simulink model "Hacheur_4_quadrant"  (R2013a)
settings: Solver=ode1  StartTime=0.0  StopTime=10  FixedStep=1e-5  RelTol=1e-3
undefined symbols (not defined in the file or in its folder): Tmli
libraries: powerlib x10, simulink x1
settings Model: Creator=hp  LastModifiedBy=hp
settings DataIOCC: InspectSignalLogs=on

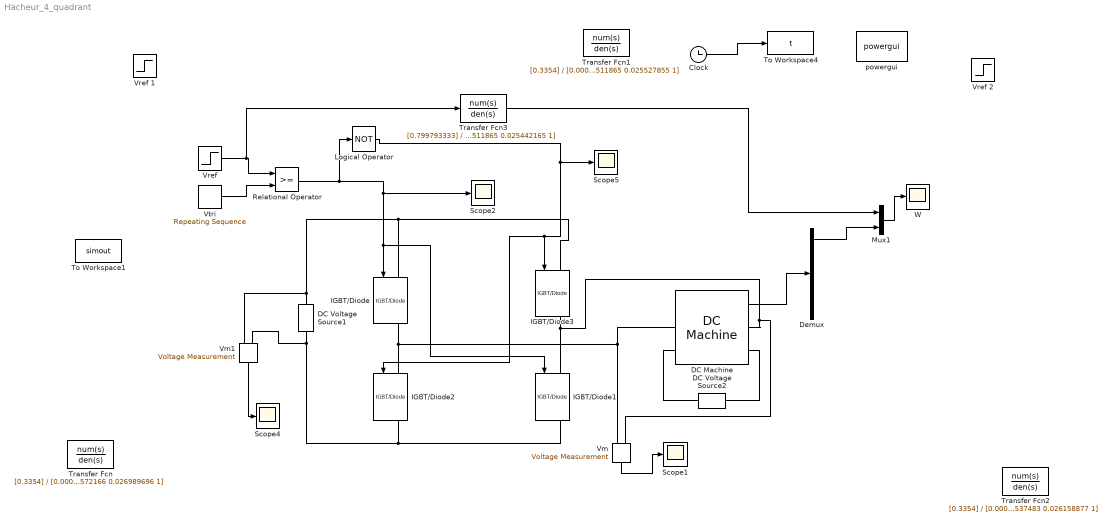
== system Hacheur_4_quadrant ==
  Clock : Clock
  DC Machine : powerlib/Machines/DC Machine  PresetModel=02: 5HP 240V 1750RPM Field:150V  MechanicalLoad=Torque TL  FieldType=Wound  ShowDetailedParameters=on  RLa=[0.78 0.016]  RLf=[150 112.5]  Laf=1.234  MachineConstant=Torque constant (N.m/A)  Ke=1.8  Kt=1.8  J=0.05  Bm=0.01  Tf=0  w0=1  Ifinit=1  TsPowergui=0  TsBlock=-1
  DC Voltage Source1 : powerlib/Electrical Sources/DC Voltage Source  Amplitude=240  Measurements=None
  DC Voltage Source2 : powerlib/Electrical Sources/DC Voltage Source  Amplitude=150  Measurements=None
  Demux : Demux
  IGBT/Diode{,1..3} (4 alike) : powerlib/Power Electronics/IGBT//Diode  Ron=1e-3  Rs=1e5  Cs=inf  Measurements=on
  Logical Operator : Logic  Operator=NOT  AllPortsSameDT=off  OutDataTypeStr=boolean
  Mux1 : Mux  Inputs=2
  Relational Operator : RelationalOperator  OutDataTypeStr=boolean
  Scope{1..2,4..5} (4 alike) : Scope
      Scope4 settings: SaveName=ScopeData3
      Scope5 settings: SaveName=ScopeData4
  To Workspace1 : ToWorkspace  VariableName=simout  SampleTime=-1  SaveFormat=Timeseries
  To Workspace4 : ToWorkspace  VariableName=t  SampleTime=-1  SaveFormat=Timeseries
  Transfer Fcn : TransferFcn  Numerator=[0.3354]  Denominator=[0.000572166 0.026989696 1]
  Transfer Fcn1 : TransferFcn  Numerator=[0.3354]  Denominator=[0.000511865 0.025527855 1]
  Transfer Fcn2 : TransferFcn  Numerator=[0.3354]  Denominator=[0.000537483 0.026158877 1]
  Transfer Fcn3 : TransferFcn  Numerator=[0.799793333]  Denominator=[0.000511865 0.025442165 1]
  Vm : powerlib/Measurements/Voltage Measurement  PhasorSimulation=off  OutputType=Complex  PSBequivalent=0
  Vm1 : powerlib/Measurements/Voltage Measurement  PhasorSimulation=off  OutputType=Complex  PSBequivalent=0
  "Vref " : Step  Time=0  After=-150  SampleTime=0
  Vref 1 : Step  Time=10  After=2  SampleTime=0
  Vref 2 : Step  Time=0  After=200  SampleTime=0
  Vtri : simulink/Sources/Repeating Sequence  rep_seq_t=[0 (1/2) 1]*Tmli  rep_seq_y="[-1  1 -1] *240"
  W : Scope
      settings: YMin=-6.7  YMax=6.7  SaveName=Vitesse
  powergui : powerlib/powergui  Priority=1  SimulationMode=Continuous  SolverType=Tustin  SampleTime=50e-6  frequency=60  SPID=off  DisableSnubberDevices=off  DisableRonSwitches=off  DisableVfSwitches=off  SwTol=0  Interpol=off  DisplayEquations=off  frequencyindice=0  Pbase=100e6  ErrMax=1e-4  Iterations=50  UnitsV=kV  UnitsW=MW  FunctionMessages=off  echomessages=off  HookPort=off  EnableUseOfTLC=off  x0status=blocks  RestoreLinks=warning  ResistiveCurrentMeasurement=off  Frange=[0:2:500]  Ylog=off  Xlog=on  ShowGrid=off  save=off  variable=ZData  ZoomFFT=off  StartTime=0.0  cycles=1  DisplayStyle=1  fundamental=60  FreqAxis=off  MaxFrequency=1000  frequencyindicesteady=1  RmsSteady=1  display=off  Ts=0  methode=off
  wires:
  Logical Operator/1 -> IGBT/Diode2/1, IGBT/Diode3/1, Scope5/1
  Relational Operator/1 -> Logical Operator/1, Scope2/1, IGBT/Diode1/1, IGBT/Diode/1
  Vm/1 -> Scope1/1
  DC Machine/1 -> Demux/1
  Clock/1 -> To Workspace4/1
  Vtri/1 -> Relational Operator/2
  Mux1/1 -> W/1
  Vm1/1 -> Scope4/1
  Demux/1 -> Mux1/2
  "Vref "/1 -> Transfer Fcn3/1, Relational Operator/1
  Transfer Fcn3/1 -> Mux1/1
  connections:
  Vm1/LConn1 -- DC Voltage Source1/RConn1 -- IGBT/Diode3/LConn1 -- IGBT/Diode/LConn1
  Vm/LConn2 -- DC Machine/RConn1 -- IGBT/Diode3/RConn1 -- IGBT/Diode1/LConn1
  DC Machine/LConn1 -- Vm/LConn1 -- IGBT/Diode/RConn1 -- IGBT/Diode2/LConn1
  IGBT/Diode2/RConn1 -- IGBT/Diode1/RConn1 -- Vm1/LConn2 -- DC Voltage Source1/LConn1
  DC Voltage Source2/LConn1 -- DC Machine/RConn2
  DC Voltage Source2/RConn1 -- DC Machine/LConn2
